simulink model "CSDProj1Q2"  (R2019b)
settings: Solver=VariableStepAuto  StartTime=0.0  StopTime=15  RelTol=1e-3
values from neighbouring files (symbols this model uses):
  A = 5e-3    (= 0.005)    [CSDProj1Q2.m]
  A_sys = double(subs(jacobian(F,X),[X_3 U_1],[x_3_star u_1_star]))    [CSDProj1Q2.m]
  B_sys = double(subs(jacobian(F,U),[X_3 U_1],[x_3_star u_1_star]))    [CSDProj1Q2.m]
  beta = 1e9    (= 1000000000)    [CSDProj1Q2.m]
  C_sys = double(jacobian(G,X))    [CSDProj1Q2.m]
  cf = 9e3    (= 9000)    [CSDProj1Q2.m]
  ct = 2e-10    [CSDProj1Q2.m]
  D_sys = double(jacobian(G,U))    [CSDProj1Q2.m]
  g = 9.81    [CSDProj1Q2.m]
  KQ = 2e-3    (= 0.002)    [CSDProj1Q2.m]
  m = 1230    [CSDProj1Q1.m]    (also in CSDProj1Q2.m = 100)
  ps = 7e6    (= 7000000)    [CSDProj1Q2.m]
  rho = 850    [CSDProj1Q2.m]
  u_1_star = ct * m * g / (KQ * A * sqrt((ps - m * g * sign(1)) / rho))    [CSDProj1Q2.m]
  u_2_star = m * g    (= 981)    [CSDProj1Q2.m]
  V = simulation_output.V(:,2)    [CSDProj1Q1.m]    (also in CSDProj1Q2.m = 0.011)
  x_3_star = m * g / A    (= 196200)    [CSDProj1Q2.m]
undefined symbols (not defined in the file or in its folder): sigbuilder_block
libraries: cstblocks x4
settings Model: Creator=shlomishetrit  LastModifiedBy=shlomishetrit

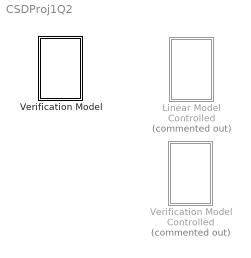
== system CSDProj1Q2 ==
  Linear Model Controlled : Subsystem  Commented=on
  Verification Model : Subsystem
  Verification Model Controlled : Subsystem  Commented=on

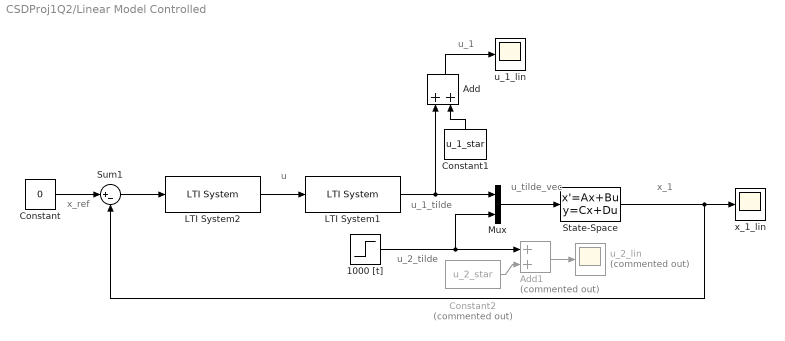
== system CSDProj1Q2/Linear Model Controlled ==
  note: u
  note: u_tilde_vec
  note: u_1
  note: u_2_tilde
  note: x_1
  note: u_1_tilde
  note: x_ref
  1000 [t] : Step  Time=0  After=1000 * g  SampleTime=0
  Add : Sum
  Add1 : Sum  Commented=on
  Constant : Constant  Value=0
  Constant1 : Constant  Value=u_1_star
  Constant2 : Constant  Commented=on  Value=u_2_star
  LTI System1 : cstblocks/LTI System  sys=G_u_xv  IC=[]
  LTI System2 : cstblocks/LTI System  sys=c  IC=[]
  Mux : Mux  Inputs=2
  State-Space : StateSpace  A=A_sys  B=B_sys  C=C_sys  D=D_sys  InitialCondition=0
  Sum1 : Sum  Inputs=|+-
  u_1_lin : Scope
  u_2_lin : Scope  Commented=on
  x_1_lin : Scope
  wires:
  Sum1/1 -> LTI System2/1
  State-Space/1 -> x_1_lin/1, Sum1/2
  LTI System2/1 -> LTI System1/1
  LTI System1/1 -> Mux/1, Add/1
  Mux/1 -> State-Space/1
  1000 [t]/1 -> Add1/1, Mux/2
  Constant/1 -> Sum1/1
  Add/1 -> u_1_lin/1
  Constant1/1 -> Add/2
  Constant2/1 -> Add1/2
  Add1/1 -> u_2_lin/1

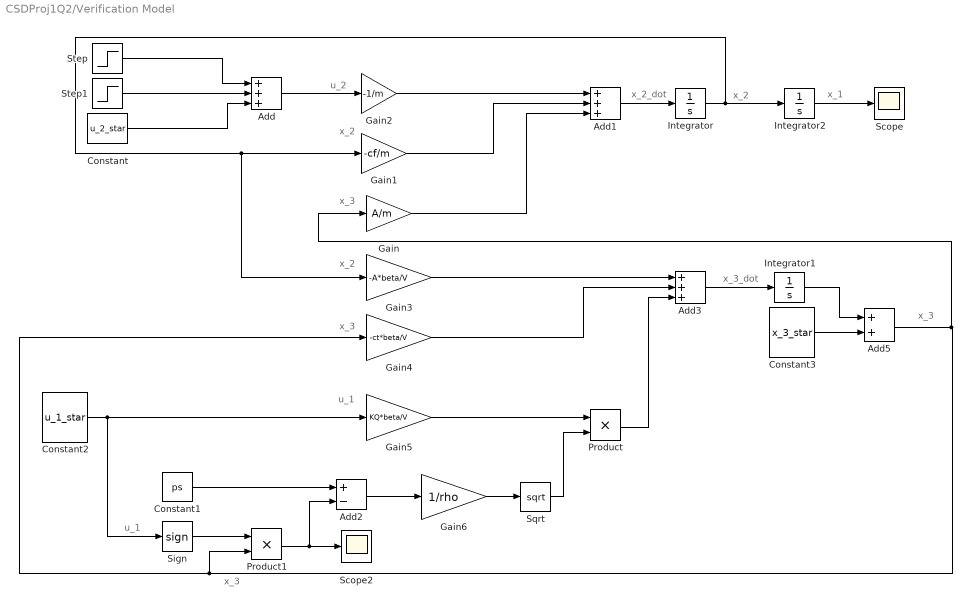
== system CSDProj1Q2/Verification Model ==
  note: x_1
  note: x_3_dot
  note: x_2_dot
  note: x_2
  note: x_3
  note: x_3
  note: u_1
  note: u_1
  note: x_2
  note: x_3
  note: x_3
  note: x_2
  note: u_2
  Add : Sum  Inputs=+++
  Add1 : Sum  Inputs=+++
  Add2 : Sum  Inputs=+-
  Add3 : Sum  Inputs=+++
  Add5 : Sum
  Constant : Constant  Value=u_2_star
  Constant1 : Constant  Value=ps
  Constant2 : Constant  Value=u_1_star
  Constant3 : Constant  Value=x_3_star
  Gain : Gain  Gain=A/m
  Gain1 : Gain  Gain=-cf/m
  Gain2 : Gain  Gain=-1/m
  Gain3 : Gain  Gain=-A*beta/V
  Gain4 : Gain  Gain=-ct*beta/V
  Gain5 : Gain  Gain=KQ*beta/V
  Gain6 : Gain  Gain=1/rho
  Integrator : Integrator
  Integrator1 : Integrator
  Integrator2 : Integrator
  Product : Product
  Product1 : Product
  Scope : Scope
  Scope2 : Scope
  Sign : Signum  ZeroCross=off
  Sqrt : Sqrt  SaturateOnIntegerOverflow=on
  Step : Step  Time=0  After=1000 * g  SampleTime=0
  Step1 : Step  Time=5  After=-1000 * g  SampleTime=0
  wires:
  Gain2/1 -> Add1/1
  Gain3/1 -> Add3/1
  Product/1 -> Add3/3
  Constant/1 -> Add/3
  Sqrt/1 -> Product/2
  Integrator1/1 -> Add5/1
  Add2/1 -> Gain6/1
  Add1/1 -> Integrator/1
  Constant1/1 -> Add2/1
  Gain1/1 -> Add1/2
  Integrator2/1 -> Scope/1
  Sign/1 -> Product1/1
  Step/1 -> Add/1
  Add/1 -> Gain2/1
  Gain5/1 -> Product/1
  Product1/1 -> Add2/2, Scope2/1
  Constant3/1 -> Add5/2
  Gain/1 -> Add1/3
  Gain4/1 -> Add3/2
  Add5/1 -> Gain4/1, Product1/2, Gain/1
  Gain6/1 -> Sqrt/1
  Add3/1 -> Integrator1/1
  Integrator/1 -> Integrator2/1, Gain3/1, Gain1/1
  Step1/1 -> Add/2
  Constant2/1 -> Sign/1, Gain5/1

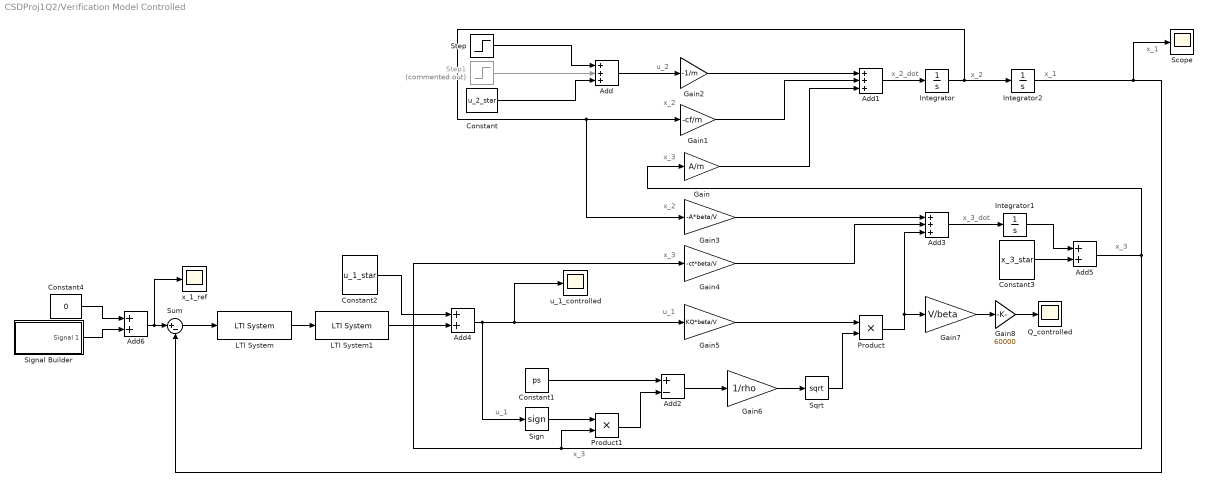
== system CSDProj1Q2/Verification Model Controlled ==
  note: x_1
  note: x_1
  note: x_3_dot
  note: x_2_dot
  note: x_2
  note: x_3
  note: x_3
  note: u_1
  note: u_1
  note: x_2
  note: x_3
  note: x_3
  note: x_2
  note: u_2
  Add : Sum  Inputs=+++
  Add1 : Sum  Inputs=+++
  Add2 : Sum  Inputs=+-
  Add3 : Sum  Inputs=+++
  Add4 : Sum
  Add5 : Sum
  Add6 : Sum
  Constant : Constant  Value=u_2_star
  Constant1 : Constant  Value=ps
  Constant2 : Constant  Value=u_1_star
  Constant3 : Constant  Value=x_3_star
  Constant4 : Constant  Value=0
  Gain : Gain  Gain=A/m
  Gain1 : Gain  Gain=-cf/m
  Gain2 : Gain  Gain=-1/m
  Gain3 : Gain  Gain=-A*beta/V
  Gain4 : Gain  Gain=-ct*beta/V
  Gain5 : Gain  Gain=KQ*beta/V
  Gain6 : Gain  Gain=1/rho
  Gain7 : Gain  Gain=V/beta
  Gain8 : Gain  Gain=60000
  Integrator : Integrator
  Integrator1 : Integrator
  Integrator2 : Integrator
  LTI System : cstblocks/LTI System  sys=c  IC=[]
  LTI System1 : cstblocks/LTI System  sys=G_u_xv  IC=[]
  Product : Product
  Product1 : Product
  Q_controlled : Scope
  Scope : Scope
  Sign : Signum  ZeroCross=off
  Signal Builder : Subsystem  Tag=STV Subsys  LoadFcn=sigbuilder_block('load');  StartFcn=sigbuilder_block('start');  StopFcn=sigbuilder_block('stop');  ClipboardFcn=sigbuilder_block('clipboard');  mask(Sigbuilder block){tuvar=[0:10]}
      mask help: Simulink:masks:SigbuilderBlock_MD
      mask init:
      | if ~strcmp(get_param(bdroot(gcbh),'SimulationStatus'),'stopped') tuvar = sigbuilder_block('maskInit'); end
      settings: CopyFcn=sigbuilder_block('copy');  DeleteFcn=sigbuilder_block('delete');  ModelCloseFcn=sigbuilder_block('modelClose');  PreSaveFcn=sigbuilder_block('preSave');  PauseFcn=sigbuilder_block('pause');  ContinueFcn=sigbuilder_block('continue');  NameChangeFcn=sigbuilder_block('namechange');  OpenFcn=sigbuilder_block('open',[437.6 199.2 550.4 400 ]);  CloseFcn=sigbuilder_block('close');
      mask Display: plot(0, 0, 100, 100,[2, 2, 32, 32, 2], [68, 8, 8, 68, 68],[32, 2], [38, 38], [32, 19, 2],[53, 60, 44], [32, 17, 17, 2],[16, 16, 31, 31]);txt = getActiveGroup(gcbh);text(2, 100, txt,'verticalAlignment', 'top');
  Sqrt : Sqrt  SaturateOnIntegerOverflow=on
  Step : Step  Time=0  After=1000 * g  SampleTime=0
  Step1 : Step  Commented=on  After=-1000 * g  SampleTime=0
  Sum : Sum  Inputs=|+-
  u_1_controlled : Scope
  x_1_ref : Scope
  wires:
  Gain2/1 -> Add1/1
  Gain3/1 -> Add3/1
  Product/1 -> Add3/3, Gain7/1
  Constant/1 -> Add/3
  Sqrt/1 -> Product/2
  Integrator1/1 -> Add5/1
  Add2/1 -> Gain6/1
  Add1/1 -> Integrator/1
  Constant1/1 -> Add2/1
  Gain1/1 -> Add1/2
  Integrator2/1 -> Scope/1, Sum/2
  Sign/1 -> Product1/1
  Step/1 -> Add/1
  Add/1 -> Gain2/1
  Gain5/1 -> Product/1
  Product1/1 -> Add2/2
  Constant3/1 -> Add5/2
  Gain/1 -> Add1/3
  Gain4/1 -> Add3/2
  Add5/1 -> Gain4/1, Product1/2, Gain/1
  Gain6/1 -> Sqrt/1
  Add3/1 -> Integrator1/1
  Integrator/1 -> Integrator2/1, Gain3/1, Gain1/1
  Step1/1 -> Add/2
  Sum/1 -> LTI System/1
  LTI System/1 -> LTI System1/1
  Add4/1 -> u_1_controlled/1, Gain5/1, Sign/1
  Constant2/1 -> Add4/1
  LTI System1/1 -> Add4/2
  Gain7/1 -> Gain8/1
  Gain8/1 -> Q_controlled/1
  Add6/1 -> x_1_ref/1, Sum/1
  Constant4/1 -> Add6/1
  Signal Builder/1(Signal 1) -> Add6/2

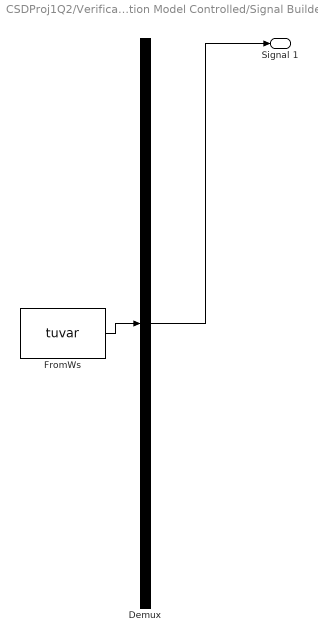
== system CSDProj1Q2/Verification Model Controlled/Signal Builder ==
  Demux : Demux  Tag=STV Demux  Outputs=1
  FromWs : FromWorkspace  Tag=STV FromWs  VariableName=tuvar  SampleTime=0
      SigBuilderData=|
      | common.afterFinalStr = 'Extrapolate'
      | common.sampleTime = 0
      | dataSet.timeRange = [0 10]
      | dataSet.name = 'Group 1'
      | sbobj.Groups.Name = 'Group 1'
      | sbobj.Groups.Signals.Name = 'Signal 1'
      | sbobj.Groups.Signals.XData = [0 1 7 10]
      | sbobj.Groups.Signals.YData = [0 0 1 1]
  Signal 1 : Outport  Tag=STV Outport
  wires:
  Demux/1 -> Signal 1/1
  FromWs/1 -> Demux/1
